simulink model "SERIALCOMM"  (R2020a)
settings: Solver=FixedStepAuto  StartTime=0.0  StopTime=10.0  FixedStep=1e-3  RelTol=1e-3  EnableMultiTasking=on
undefined symbols (not defined in the file): A0, A1, PTB2, PTB3
libraries: frdmk64flib x8, etargetslib x2
settings Model: ExtModeTrigDuration=5  Creator=Nour  LastModifiedBy=Nour
settings OptimizationCC: EnhancedBackFolding=on  PassReuseOutputArgsAs=Individual arguments  ZeroExternalMemoryAtStartup=off  ZeroInternalMemoryAtStartup=off  MaxStackSize=64  OptimizeBlockOrder=speed  DifferentSizesBufferReuse=on  OptimizationCustomize=off  EfficientTunableParamExpr=on
settings DebuggingCC: ParameterTunabilityLossMsg=error
settings HardwareCC: ProdBitPerPointer=32  ProdBitPerSizeT=32  ProdBitPerPtrDiffT=32  ProdLargestAtomicInteger=Long  ProdLargestAtomicFloat=Double  ProdWordSize=32  ProdHWDeviceType=ARM Compatible->ARM Cortex
settings SFSimCC: MATLABDynamicMemAlloc=off
settings RTWCC: SystemTargetFile=ert.tlc  HardwareBoard=NXP FRDM-K64F  TemplateMakefile=ert_default_tmf  Toolchain=GNU Tools for ARM Embedded Processors
settings CodeAppCC: ForceParamTrailComments=on  IgnoreCustomStorageClasses=off  OperatorAnnotations=on  SimulinkDataObjDesc=on  SFDataObjDesc=on  InsertBlockDesc=on

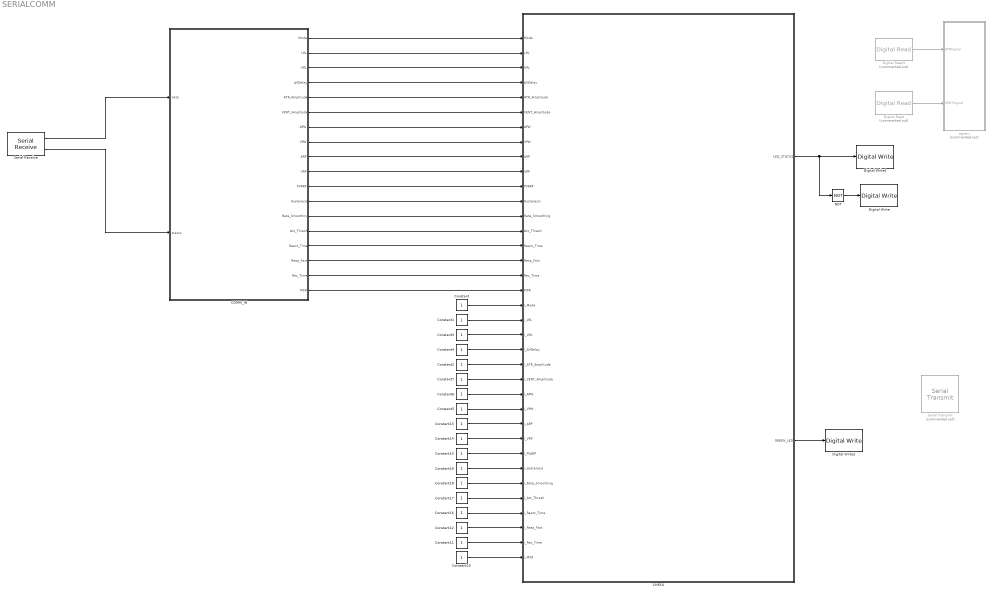
== system SERIALCOMM ==
  CHECK : Stateflow chart  TreatAsAtomicUnit=on
  COMM_IN : Stateflow chart  TreatAsAtomicUnit=on
  Constant{,1..3,5..7,10..12,16..19} (14 alike) : Constant  OutDataTypeStr=uint8
  Constant{4,13..15} (4 alike) : Constant  OutDataTypeStr=uint16
  Digital Read : frdmk64flib/Digital Read  Commented=on  Whichpin=PTB3 (A1)  SampleTime=-1
  Digital Read1 : frdmk64flib/Digital Read  Commented=on  Whichpin=PTB2 (A0)  SampleTime=-1
  Digital Write : frdmk64flib/Digital Write  Whichpin=RED_LED
  Digital Write1 : frdmk64flib/Digital Write  Whichpin=BLUE_LED
  Digital Write2 : frdmk64flib/Digital Write  Whichpin=GREEN_LED
  NOT : Logic  Operator=NOT  IconShape=distinctive  AllPortsSameDT=off  OutDataTypeStr=boolean
  Serial Receive : frdmk64flib/Serial Receive  SCIModule=0  Baudrate=uint32(9600)  Parity=None  StopBits=1  HardwareFlowControl=None  ByteOrder=LittleEndian  DataType=uint8  DataLength=30  BlockingMode=off  OutputStatus=on  SampleTime=-1
  Serial Transmit : frdmk64flib/Serial Transmit  Commented=on  SCIModule=0  Baudrate=uint32(9600)  Parity=None  StopBits=1  HardwareFlowControl=None  ByteOrder=LittleEndian  BlockingMode=on  OutputStatus=off
  egram : Subsystem  Commented=on
  wires:
  Serial Receive/1 -> COMM_IN/1(data)
  Serial Receive/2 -> COMM_IN/2(status)
  Digital Read/1 -> egram/2(VENTSignal)
  Digital Read1/1 -> egram/1(ATRSignal)
  CHECK/2(GREEN_LED) -> Digital Write2/1
  NOT/1 -> Digital Write/1
  CHECK/1(LED_STATUS) -> Digital Write1/1, NOT/1
  Constant/1 -> CHECK/19(i_Mode)
  Constant1/1 -> CHECK/20(i_LRL)
  Constant3/1 -> CHECK/21(i_URL)
  Constant4/1 -> CHECK/22(i_AVDelay)
  Constant2/1 -> CHECK/23(i_ATR_Amplitude)
  Constant7/1 -> CHECK/24(i_VENT_Amplitude)
  Constant6/1 -> CHECK/25(i_APW)
  Constant5/1 -> CHECK/26(i_VPW)
  Constant15/1 -> CHECK/27(i_ARP)
  Constant14/1 -> CHECK/28(i_VRP)
  Constant13/1 -> CHECK/29(i_PVARP)
  Constant19/1 -> CHECK/30(i_Hysteresis)
  Constant18/1 -> CHECK/31(i_Rate_Smoothing)
  Constant17/1 -> CHECK/32(i_Act_Thresh)
  Constant16/1 -> CHECK/33(i_React_Time)
  Constant12/1 -> CHECK/34(i_Resp_Fact)
  Constant11/1 -> CHECK/35(i_Rec_Time)
  Constant10/1 -> CHECK/36(i_MSR)
  COMM_IN/1(Mode) -> CHECK/1(Mode)
  COMM_IN/2(LRL) -> CHECK/2(LRL)
  COMM_IN/3(URL) -> CHECK/3(URL)
  COMM_IN/4(AVDelay) -> CHECK/4(AVDelay)
  COMM_IN/5(ATR_Amplitude) -> CHECK/5(ATR_Amplitude)
  COMM_IN/6(VENT_Amplitude) -> CHECK/6(VENT_Amplitude)
  COMM_IN/7(APW) -> CHECK/7(APW)
  COMM_IN/8(VPW) -> CHECK/8(VPW)
  COMM_IN/9(ARP) -> CHECK/9(ARP)
  COMM_IN/10(VRP) -> CHECK/10(VRP)
  COMM_IN/11(PVARP) -> CHECK/11(PVARP)
  COMM_IN/12(Hysteresis) -> CHECK/12(Hysteresis)
  COMM_IN/13(Rate_Smoothing) -> CHECK/13(Rate_Smoothing)
  COMM_IN/14(Act_Thresh) -> CHECK/14(Act_Thresh)
  COMM_IN/15(React_Time) -> CHECK/15(React_Time)
  COMM_IN/18(MSR) -> CHECK/18(MSR)
  COMM_IN/17(Rec_Time) -> CHECK/17(Rec_Time)
  COMM_IN/16(Resp_Fact) -> CHECK/16(Resp_Fact)

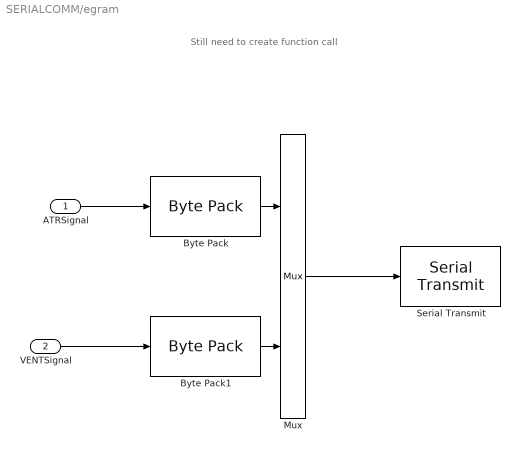
== system SERIALCOMM/egram ==
  note: Still need to create function call
  ATRSignal : Inport
  VENTSignal : Inport  Port=2
  Byte Pack : etargetslib/Byte Pack  datatypes={'double'}  byteAlign=1
  Byte Pack1 : etargetslib/Byte Pack  datatypes={'double'}  byteAlign=1
  Mux : Mux  Inputs=2
  Serial Transmit : frdmk64flib/Serial Transmit  SCIModule=0  Baudrate=uint32(9600)  Parity=None  StopBits=1  HardwareFlowControl=None  ByteOrder=LittleEndian  BlockingMode=on  OutputStatus=off
  wires:
  ATRSignal/1 -> Byte Pack/1
  Byte Pack1/1 -> Mux/2
  Byte Pack/1 -> Mux/1
  VENTSignal/1 -> Byte Pack1/1
  Mux/1 -> Serial Transmit/1

== stateflow chart SERIALCOMM/COMM_IN ==
  state SET_PARAM
    %% setting parameter values through
    %% serial communication
    Mode = typecast(data(3), 'uint8');
    URL = typecast(data(4), 'uint8');
    LRL = typecast(data(5), 'uint8');
    VENT_Amplitude = typecast(data(6), 'uint8');
    VPW = typecast(data(7), 'uint8');
    ATR_Amplitude = typecast(data(8), 'uint8');
    APW = typecast(data(9), 'uint8');
    VRP = typecast(data(10:11), 'uint16');
    ARP = typecast(data(12:13), 'uint16');
    PVARP = typecast(data(14:15), 'uint16');
    Hysteresis = typecast(data(16), 'uint8');
    Rate_Smoothing = typecast(data(17), 'uint8');
    AVDelay = typecast(data(18: 19), 'uint16');
    MSR = typecast(data(20), 'uint8');
    Act_Thresh = typecast(data(21), 'uint8');
    React_Time = typecast(data(22), 'uint8');
    Resp_Fact = typecast(data(23), 'uint8');
    Rec_Time = typecast(data(24), 'uint8');
  state INITIAL
    %% Setting initial, default values of parameters
    entry:
    Mode = 0;
    URL = 0;
    LRL = 0;
    VENT_Amplitude = 0;
    VPW = 0;
    ATR_Amplitude = 0;
    APW = 0;
    VRP = 0;
    ARP = 0;
    PVARP = 0;
    Hysteresis = 0;
    Rate_Smoothing = 0;
    AVDelay = 0;
    MSR = 0;
    Act_Thresh = 0;
    React_Time = 0;
    Resp_Fact = 0;
    Rec_Time = 0;
  state STANDBY
    %% Waiting for COM
  state ECHO_PARAM
    entry:
    %%send_params();
  (junction 15) -> SET_PARAM [order 2] : [data(2) == hex2dec('55')]
  SET_PARAM -> STANDBY
  (default) -> INITIAL
  (junction 13) -> STANDBY [order 2]
  INITIAL -> STANDBY
  STANDBY -> (junction 13) [order 1] : [status == 0]
  (junction 13) -> (junction 15) [order 1] : [data(1) == hex2dec('16')]
  (junction 15) -> ECHO_PARAM [order 1] : [status == 0]
  ECHO_PARAM -> STANDBY : [status == 32]
  STANDBY -> ECHO_PARAM [order 2] : [status == 32]
  data: data input uint8 size=[30;1]; status input uint8 size=[1;1]; Mode output uint8; LRL output uint8; URL output uint8; AVDelay output uint16; ATR_Amplitude output uint8; VENT_Amplitude output uint8; APW output uint8; VPW output uint8; ARP output uint16; VRP output uint16; PVARP output uint16; Hysteresis output uint8; Rate_Smoothing output uint8; Act_Thresh output uint8; React_Time output uint8; Resp_Fact output uint8; Rec_Time output uint8; MSR output uint8

== stateflow chart SERIALCOMM/CHECK ==
  state ENTRY
    %% @Matt, you need to enter the values here:
    %% replace the 00's with your values
    entry:
    GREEN_LED = true;
  state URLCheck
    entry:
    LED_STATUS = (URL == i_URL);
  state AVDelayCheck
    entry:
    LED_STATUS = (AVDelay == i_AVDelay);
  state ATR_ACheck
    entry:
    LED_STATUS = (ATR_Amplitude == i_ATR_Amplitude);
  state ModeCheck
    entry:
    LED_STATUS = (Mode == i_Mode);
  state LRLCheck
    entry:
    LED_STATUS = (LRL == i_LRL);
  state VENT_ACheck
    entry:
    LED_STATUS = (VENT_Amplitude == i_VENT_Amplitude);
  state VRPCheck
    entry:
    LED_STATUS = (VRP == i_VRP);
  state ARPCheck
    entry:
    LED_STATUS = (ARP == i_ARP);
  state APWCheck
    entry:
    LED_STATUS = (APW == i_APW);
  state VPWCheck
    entry:
    LED_STATUS = (VPW == i_VPW);
  state React_TimeCheck
    entry:
    LED_STATUS = (React_Time == i_React_Time);
  state PVARPCheck
    entry:
    LED_STATUS = (PVARP == i_PVARP);
  state HystCheck
    entry:
    LED_STATUS = (Hysteresis == i_Hysteresis);
  state Act_ThreshCheck
    entry:
    LED_STATUS = (Act_Thresh == i_Act_Thresh);
  state Rate_SmoothCheck
    entry:
    LED_STATUS = (Rate_Smoothing == i_Rate_Smoothing);
  state MSRCheck
    entry:
    LED_STATUS = (MSR == i_MSR);
  state Rec_TimeCheck
    entry:
    LED_STATUS = (Rec_Time == i_Rec_Time);
  state Resp_FactCheck
    entry:
    LED_STATUS = (Resp_Fact == i_Resp_Fact);
  (default) -> ENTRY
  URLCheck -> AVDelayCheck : [after(1000, msec)]
  LRLCheck -> URLCheck : [after(1000, msec)]
  ENTRY -> ModeCheck : [after(1000, msec)]{GREEN_LED = false}
  ModeCheck -> LRLCheck : [after(1000, msec)]
  AVDelayCheck -> ATR_ACheck : [after(1000, msec)]
  MSRCheck -> ENTRY : [after(1000, msec)]
  ATR_ACheck -> VENT_ACheck : [after(1000, msec)]
  ARPCheck -> VRPCheck : [after(1000, msec)]
  VENT_ACheck -> APWCheck : [after(1000, msec)]
  VPWCheck -> ARPCheck : [after(1000, msec)]
  APWCheck -> VPWCheck : [after(1000, msec)]
  VRPCheck -> PVARPCheck : [after(1000, msec)]
  PVARPCheck -> HystCheck : [after(1000, msec)]
  Act_ThreshCheck -> React_TimeCheck : [after(1000, msec)]
  HystCheck -> Rate_SmoothCheck : [after(1000, msec)]
  Rate_SmoothCheck -> Act_ThreshCheck : [after(1000, msec)]
  React_TimeCheck -> Resp_FactCheck : [after(1000, msec)]
  Resp_FactCheck -> Rec_TimeCheck : [after(1000, msec)]
  Rec_TimeCheck -> MSRCheck : [after(1000, msec)]
  data: Mode input uint8; LRL input uint8; URL input uint8; AVDelay input uint16; ATR_Amplitude input uint8; VENT_Amplitude input uint8; APW input uint8; VPW input uint8; ARP input uint16; VRP input uint16; PVARP input uint16; Hysteresis input uint8; Rate_Smoothing input uint8; Act_Thresh input uint8; React_Time input uint8; Resp_Fact input uint8; Rec_Time input uint8; MSR input uint8; LED_STATUS output boolean; GREEN_LED output boolean; i_Mode input uint8; i_LRL input uint8; i_URL input uint8; i_AVDelay input uint16; i_ATR_Amplitude input uint8; i_VENT_Amplitude input uint8; i_APW input uint8; i_VPW input uint8; i_ARP input uint16; i_VRP input uint16; i_PVARP input uint16; i_Hysteresis input uint8; i_Rate_Smoothing input uint8; i_Act_Thresh input uint8; i_React_Time input uint8; i_Resp_Fact input uint8; i_Rec_Time input uint8; i_MSR input uint8
